simulink model "chap8_1sim"  (Simulink 5.0)
settings: Solver=ode45  StartTime=0.0  StopTime=20  FixedStep=0.001  RelTol=1e-3
settings Model: LastModifiedBy=Administrator  ExtModeTrigMode=oneshot  ExtModeArmWhenConnect=off  LimitDataPoints=off  BooleanDataType=off

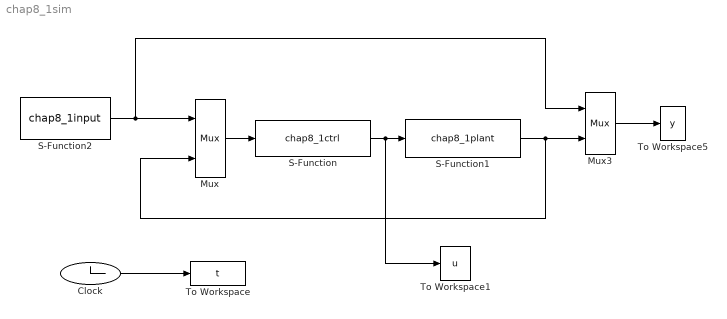
== system chap8_1sim ==
  Clock : Clock
  Mux : Mux  Inputs=2
  Mux3 : Mux  Inputs=2
  S-Function : S-Function  FunctionName=chap8_1ctrl
  S-Function1 : S-Function  FunctionName=chap8_1plant
  S-Function2 : S-Function  FunctionName=chap8_1input
  To Workspace : ToWorkspace  VariableName=t  SampleTime=-1  SaveFormat=Array
  To Workspace1 : ToWorkspace  VariableName=u  SampleTime=-1  SaveFormat=Array
  To Workspace5 : ToWorkspace  VariableName=y  SampleTime=-1  SaveFormat=Array
  wires:
  Mux/1 -> S-Function/1
  Mux3/1 -> To Workspace5/1
  S-Function/1 -> S-Function1/1, To Workspace1/1
  S-Function1/1 -> Mux/2, Mux3/2
  S-Function2/1 -> Mux/1, Mux3/1
  Clock/1 -> To Workspace/1
